simulink model "SDV"  (R2017a)
settings: Solver=ode4  StartTime=0.0  StopTime=100  FixedStep=0.01  RelTol=1e-3
values from neighbouring files (symbols this model uses):
  b = 0.1    [sdv_motion_control.m]
  d_stpms = 0.2    [sdv_motion_control.m]
  J = 0.01    [sdv_motion_control.m]
  ka = 5.0    (= 5)    [sdv_motion_control.m]
  kb = 5.0    (= 5)    [sdv_motion_control.m]
  ke = 0.1    [sdv_motion_control.m]
  kt = 0.1    [sdv_motion_control.m]
  L = 0.5    [sdv_motion_control.m]
  mod_engranajes = 0.5    [sdv_motion_control.m]
  R = 1.0    (= 1)    [sdv_motion_control.m]
  r_rueda = 0.025    [sdv_motion_control.m]
  thresh_ang = 30*pi/180    (= 0.523598775598)    [sdv_motion_control.m]
  v_max = 18    [sdv_motion_control.m]
libraries: simulink x3
settings Model: Creator=Usuario  LastModifiedBy=Usuario

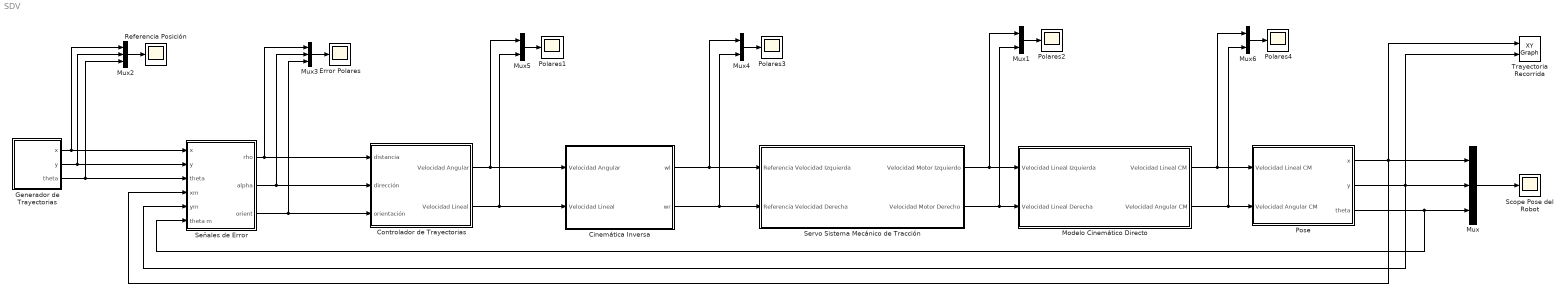
== system SDV ==
  Cinemática Inversa : Subsystem
  Controlador de Trayectorias : Subsystem
  Error Polares : Scope
  Generador de Trayectorias : Subsystem
  Modelo Cinemático Directo : Subsystem
  Mux : Mux  Inputs=3
  Mux{1,4..6} (4 alike) : Mux  Inputs=2
  Mux2 : Mux  Inputs=3
  Mux3 : Mux  Inputs=3
  Polares{1..4} (4 alike) : Scope
  Pose : Subsystem
  Referencia Posición : Scope
  Scope Pose del Robot : Scope
  Servo Sistema Mecánico de Tracción : Subsystem
  Señales de Error : Subsystem
  Trayectoria Recorrida : simulink/Sinks/XY Graph  xmin=-25  xmax=25  ymin=-25  ymax=25  st=-1
  wires:
  Mux/1 -> Scope Pose del Robot/1
  Pose/2(y) -> Trayectoria Recorrida/2, Mux/2, Señales de Error/5(ym)
  Pose/3(theta) -> Mux/3, Señales de Error/6(theta m)
  Pose/1(x) -> Trayectoria Recorrida/1, Mux/1, Señales de Error/4(xm)
  Mux2/1 -> Referencia Posición/1
  Mux3/1 -> Error Polares/1
  Mux5/1 -> Polares1/1
  Controlador de Trayectorias/1(Velocidad Angular) -> Mux5/1, Cinemática Inversa/1(Velocidad Angular)
  Señales de Error/2(alpha) -> Mux3/2, Controlador de Trayectorias/2(dirección)
  Señales de Error/1(rho) -> Mux3/1, Controlador de Trayectorias/1(distancia)
  Generador de Trayectorias/1(x) -> Mux2/1, Señales de Error/1(x)
  Generador de Trayectorias/2(y) -> Mux2/2, Señales de Error/2(y)
  Generador de Trayectorias/3(theta) -> Mux2/3, Señales de Error/3(theta)
  Señales de Error/3(orient) -> Controlador de Trayectorias/3(orientación), Mux3/3
  Controlador de Trayectorias/2(Velocidad Lineal) -> Mux5/2, Cinemática Inversa/2(Velocidad Lineal)
  Servo Sistema Mecánico de Tracción/1(Velocidad Motor Izquierdo) -> Mux1/1, Modelo Cinemático Directo/1(Velocidad Lineal Izquierda)
  Servo Sistema Mecánico de Tracción/2(Velocidad Motor Derecho) -> Mux1/2, Modelo Cinemático Directo/2(Velocidad Lineal Derecha)
  Mux1/1 -> Polares2/1
  Cinemática Inversa/1(wl) -> Mux4/1, Servo Sistema Mecánico de Tracción/1(Referencia Velocidad Izquierda)
  Mux4/1 -> Polares3/1
  Cinemática Inversa/2(wr) -> Mux4/2, Servo Sistema Mecánico de Tracción/2(Referencia Velocidad Derecha)
  Modelo Cinemático Directo/2(Velocidad Angular CM) -> Mux6/2, Pose/2(Velocidad Angular CM)
  Modelo Cinemático Directo/1(Velocidad Lineal CM) -> Mux6/1, Pose/1(Velocidad Lineal CM)
  Mux6/1 -> Polares4/1

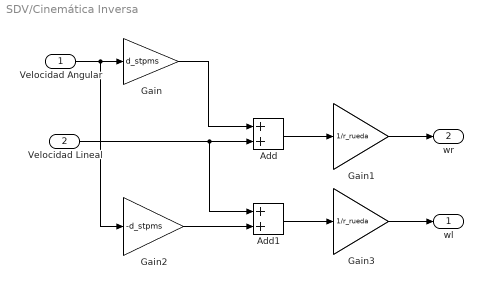
== system SDV/Cinemática Inversa ==
  Velocidad Angular : Inport
  Velocidad Lineal : Inport  Port=2
  Add : Sum
  Add1 : Sum
  Gain : Gain  Gain=d_stpms
  Gain1 : Gain  Gain=1/r_rueda
  Gain2 : Gain  Gain=-d_stpms
  Gain3 : Gain  Gain=1/r_rueda
  wl : Outport
  wr : Outport  Port=2
  wires:
  Velocidad Angular/1 -> Gain2/1, Gain/1
  Gain/1 -> Add/1
  Add/1 -> Gain1/1
  Gain1/1 -> wr/1
  Gain2/1 -> Add1/2
  Velocidad Lineal/1 -> Add1/1, Add/2
  Add1/1 -> Gain3/1
  Gain3/1 -> wl/1

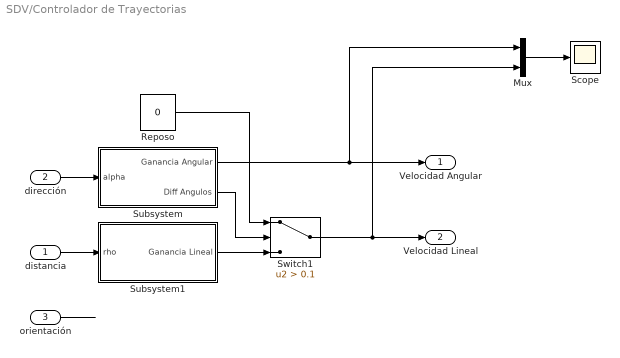
== system SDV/Controlador de Trayectorias ==
  distancia : Inport
  dirección : Inport  Port=2
  orientación : Inport  Port=3
  Mux : Mux  Inputs=2
  Reposo : Constant  Value=0
  Scope : Scope
  Subsystem : Subsystem
  Subsystem1 : Subsystem
  Switch1 : Switch  Criteria=u2 > Threshold  Threshold=0.1
  Velocidad Angular : Outport
  Velocidad Lineal : Outport  Port=2
  wires:
  dirección/1 -> Subsystem/1(alpha)
  distancia/1 -> Subsystem1/1(rho)
  Subsystem1/1(Ganancia Lineal) -> Switch1/3
  Reposo/1 -> Switch1/1
  Subsystem/2(Diff Angulos) -> Switch1/2
  Switch1/1 -> Mux/2, Velocidad Lineal/1
  Subsystem/1(Ganancia Angular) -> Mux/1, Velocidad Angular/1
  orientación/1 -> ?
  Mux/1 -> Scope/1

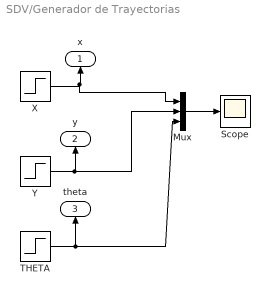
== system SDV/Generador de Trayectorias ==
  Mux : Mux  Inputs=3
  Scope : Scope
  THETA : Step  Time=0  After=0  SampleTime=0
  X : Step  Time=0  SampleTime=0
  Y : Step  Time=0  SampleTime=0
  x : Outport
  y : Outport  Port=2
  theta : Outport  Port=3
  wires:
  Y/1 -> y/1, Mux/2
  X/1 -> Mux/1, x/1
  THETA/1 -> Mux/3, theta/1
  Mux/1 -> Scope/1

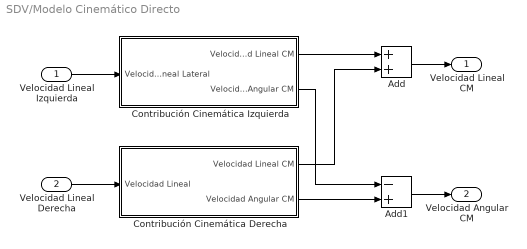
== system SDV/Modelo Cinemático Directo ==
  Velocidad Lineal Izquierda : Inport
  Velocidad Lineal Derecha : Inport  Port=2
  Add : Sum
  Add1 : Sum  Inputs=-+
  Contribución Cinemática Derecha : Subsystem
  Contribución Cinemática Izquierda : Subsystem
  Velocidad Lineal CM : Outport
  Velocidad Angular CM : Outport  Port=2
  wires:
  Velocidad Lineal Derecha/1 -> Contribución Cinemática Derecha/1(Velocidad Lineal)
  Velocidad Lineal Izquierda/1 -> Contribución Cinemática Izquierda/1(Velocidad Lineal Lateral)
  Add/1 -> Velocidad Lineal CM/1
  Add1/1 -> Velocidad Angular CM/1
  Contribución Cinemática Izquierda/2(Velocidad Angular CM) -> Add1/1
  Contribución Cinemática Derecha/2(Velocidad Angular CM) -> Add1/2
  Contribución Cinemática Derecha/1(Velocidad Lineal CM) -> Add/2
  Contribución Cinemática Izquierda/1(Velocidad Lineal CM) -> Add/1

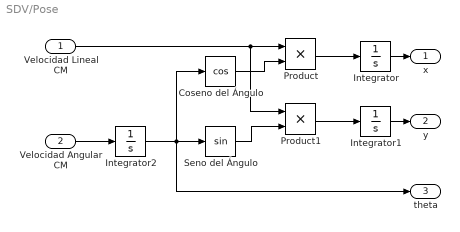
== system SDV/Pose ==
  Velocidad Lineal CM : Inport
  Velocidad Angular CM : Inport  Port=2
  Coseno del Ángulo : Trigonometry  Operator=cos
  Integrator : Integrator
  Integrator1 : Integrator
  Integrator2 : Integrator
  Product : Product
  Product1 : Product
  Seno del Ángulo : Trigonometry
  x : Outport
  y : Outport  Port=2
  theta : Outport  Port=3
  wires:
  Coseno del Ángulo/1 -> Product/2
  Integrator/1 -> x/1
  Product/1 -> Integrator/1
  Product1/1 -> Integrator1/1
  Integrator1/1 -> y/1
  Seno del Ángulo/1 -> Product1/2
  Velocidad Lineal CM/1 -> Product1/1, Product/1
  Velocidad Angular CM/1 -> Integrator2/1
  Integrator2/1 -> theta/1, Seno del Ángulo/1, Coseno del Ángulo/1

== system SDV/Servo Sistema Mecánico de Tracción ==
  Referencia Velocidad Izquierda : Inport
  Referencia Velocidad Derecha : Inport  Port=2
  Servo Controlador ESCON 50/5 Derecho : Subsystem
  Servo Controlador ESCON 50/5 Izquierdo : Subsystem
  Velocidad Motor Izquierdo : Outport
  Velocidad Motor Derecho : Outport  Port=2
  wires:
  Referencia Velocidad Izquierda/1 -> Servo Controlador ESCON 50/5 Izquierdo/1(Referencia Velocidad Izquierda)
  Referencia Velocidad Derecha/1 -> Servo Controlador ESCON 50/5 Derecho/1(Referencia Velocidad Derecha)
  Servo Controlador ESCON 50/5 Izquierdo/1(Velocidad Izquierda) -> Velocidad Motor Izquierdo/1
  Servo Controlador ESCON 50/5 Derecho/1(Velocidad Izquierda) -> Velocidad Motor Derecho/1

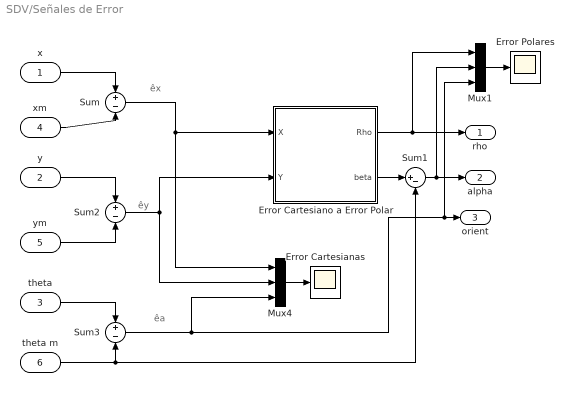
== system SDV/Señales de Error ==
  note: êa
  note: êy
  note: êx
  x : Inport
  y : Inport  Port=2
  theta : Inport  Port=3
  xm : Inport  Port=4
  ym : Inport  Port=5
  theta m : Inport  Port=6
  Error Cartesianas : Scope
  Error Polares : Scope
  Error Cartesiano a Error Polar : Subsystem
  Mux1 : Mux  Inputs=3
  Mux4 : Mux  Inputs=3
  Sum : Sum  Inputs=+-
  Sum1 : Sum  Inputs=|+-
  Sum2 : Sum  Inputs=+-
  Sum3 : Sum  Inputs=+-
  rho : Outport
  alpha : Outport  Port=2
  orient : Outport  Port=3
  wires:
  Sum/1 -> Mux4/1, Error Cartesiano a Error Polar/1(X)
  Sum2/1 -> Mux4/2, Error Cartesiano a Error Polar/2(Y)
  Error Cartesiano a Error Polar/1(Rho) -> Mux1/1, rho/1
  Mux4/1 -> Error Cartesianas/1
  Sum1/1 -> Mux1/2, alpha/1
  x/1 -> Sum/1
  y/1 -> Sum2/1
  xm/1 -> Sum/2
  ym/1 -> Sum2/2
  theta m/1 -> Sum1/2, Sum3/2
  theta/1 -> Sum3/1
  Sum3/1 -> Mux1/3, orient/1, Mux4/3
  Mux1/1 -> Error Polares/1
  Error Cartesiano a Error Polar/2(beta) -> Sum1/1

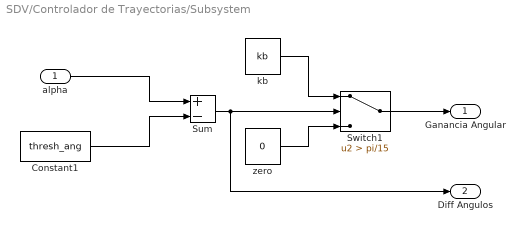
== system SDV/Controlador de Trayectorias/Subsystem ==
  alpha : Inport
  Constant1 : Constant  Value=thresh_ang
  Sum : Sum  Inputs=+-
  Switch1 : Switch  Criteria=u2 > Threshold  Threshold=pi/15
  "kb " : Constant  Value=kb
  zero : Constant  Value=0
  Ganancia Angular : Outport
  Diff Angulos : Outport  Port=2
  wires:
  Switch1/1 -> Ganancia Angular/1
  alpha/1 -> Sum/1
  Constant1/1 -> Sum/2
  "kb "/1 -> Switch1/1
  zero/1 -> Switch1/3
  Sum/1 -> Diff Angulos/1, Switch1/2

== system SDV/Controlador de Trayectorias/Subsystem1 ==
  rho : Inport
  Reposo : Constant  Value=0
  Switch : Switch  Criteria=u2 > Threshold  Threshold=0.1
  "ka " : Constant  Value=ka
  Ganancia Lineal : Outport
  wires:
  "ka "/1 -> Switch/1
  Switch/1 -> Ganancia Lineal/1
  rho/1 -> Switch/2
  Reposo/1 -> Switch/3

== system SDV/Modelo Cinemático Directo/Contribución Cinemática Derecha ==
  Velocidad Lineal : Inport
  Velcidad Lineal CM : Gain  Gain=0.5
  Velcidad Lineal CM1 : Gain  Gain=d_stpms/2
  Velocidad Lineal CM : Outport
  Velocidad Angular CM : Outport  Port=2
  wires:
  Velocidad Lineal/1 -> Velcidad Lineal CM1/1, Velcidad Lineal CM/1
  Velcidad Lineal CM/1 -> Velocidad Lineal CM/1
  Velcidad Lineal CM1/1 -> Velocidad Angular CM/1

== system SDV/Modelo Cinemático Directo/Contribución Cinemática Izquierda ==
  Velocidad Lineal Lateral : Inport
  Interpolación Lineal Angular : Gain  Gain=d_stpms/2
  Interpolación Lineal Lineal : Gain  Gain=0.5
  Velocidad Lineal CM : Outport
  Velocidad Angular CM : Outport  Port=2
  wires:
  Velocidad Lineal Lateral/1 -> Interpolación Lineal Angular/1, Interpolación Lineal Lineal/1
  Interpolación Lineal Lineal/1 -> Velocidad Lineal CM/1
  Interpolación Lineal Angular/1 -> Velocidad Angular CM/1

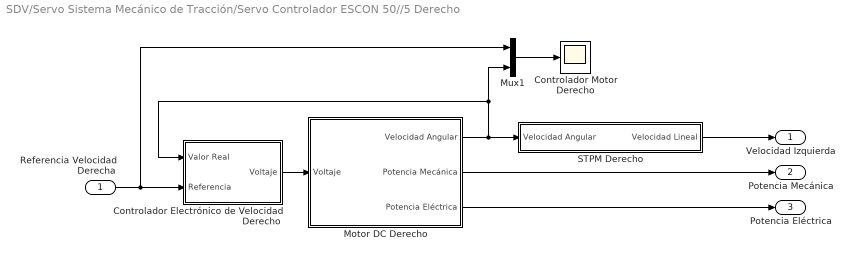
== system SDV/Servo Sistema Mecánico de Tracción/Servo Controlador ESCON 50//5 Derecho ==
  Referencia Velocidad Derecha : Inport
  Controlador Electrónico de Velocidad Derecho : Subsystem
  Controlador Motor Derecho : Scope
  Motor DC Derecho : Subsystem
  Mux1 : Mux  Inputs=2
  STPM Derecho : Subsystem
  Velocidad Izquierda : Outport
  Potencia Mecánica : Outport  Port=2
  Potencia Eléctrica : Outport  Port=3
  wires:
  Motor DC Derecho/1(Velocidad Angular) -> Mux1/2, Controlador Electrónico de Velocidad Derecho/1(Valor Real), STPM Derecho/1(Velocidad Angular)
  STPM Derecho/1(Velocidad Lineal) -> Velocidad Izquierda/1
  Controlador Electrónico de Velocidad Derecho/1(Voltaje) -> Motor DC Derecho/1("Voltaje ")
  Mux1/1 -> Controlador Motor Derecho/1
  Motor DC Derecho/2(Potencia Mecánica) -> Potencia Mecánica/1
  Motor DC Derecho/3(Potencia Eléctrica) -> Potencia Eléctrica/1
  Referencia Velocidad Derecha/1 -> Mux1/1, Controlador Electrónico de Velocidad Derecho/2(Referencia)

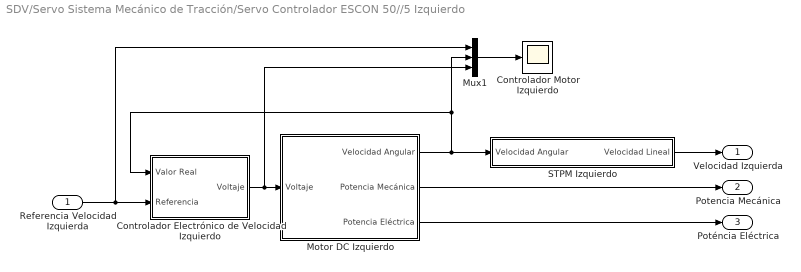
== system SDV/Servo Sistema Mecánico de Tracción/Servo Controlador ESCON 50//5 Izquierdo ==
  Referencia Velocidad Izquierda : Inport
  Controlador Electrónico de Velocidad Izquierdo : Subsystem
  Controlador Motor Izquierdo : Scope
  "Motor DC Izquierdo " : Subsystem
  Mux1 : Mux  Inputs=3
  STPM Izquierdo : Subsystem
  Velocidad Izquierda : Outport
  Potencia Mecánica : Outport  Port=2
  Poténcia Eléctrica : Outport  Port=3
  wires:
  Referencia Velocidad Izquierda/1 -> Mux1/1, Controlador Electrónico de Velocidad Izquierdo/2(Referencia)
  Controlador Electrónico de Velocidad Izquierdo/1(Voltaje) -> Mux1/3, "Motor DC Izquierdo "/1("Voltaje ")
  STPM Izquierdo/1(Velocidad Lineal) -> Velocidad Izquierda/1
  "Motor DC Izquierdo "/2(Potencia Mecánica) -> Potencia Mecánica/1
  "Motor DC Izquierdo "/3(Potencia Eléctrica) -> Poténcia Eléctrica/1
  Mux1/1 -> Controlador Motor Izquierdo/1
  "Motor DC Izquierdo "/1(Velocidad Angular) -> STPM Izquierdo/1(Velocidad Angular), Mux1/2, Controlador Electrónico de Velocidad Izquierdo/1(Valor Real)

== system SDV/Señales de Error/Error Cartesiano a Error Polar ==
  X : Inport
  Y : Inport  Port=2
  Error Cartesianas : Scope
  Mux4 : Mux  Inputs=3
  Norma Euclidea : Subsystem
  Ángulo : Trigonometry  Operator=atan2
  Rho : Outport
  beta : Outport  Port=2
  wires:
  X/1 -> Mux4/2, Ángulo/2, Norma Euclidea/1(x)
  Y/1 -> Mux4/1, Ángulo/1, Norma Euclidea/2(y)
  Ángulo/1 -> Mux4/3, beta/1
  Norma Euclidea/1(rho) -> Rho/1
  Mux4/1 -> Error Cartesianas/1

== system SDV/Servo Sistema Mecánico de Tracción/Servo Controlador ESCON 50//5 Derecho/Controlador Electrónico de Velocidad Derecho ==
  Valor Real : Inport
  Referencia : Inport  Port=2
  PID Controller : simulink/Continuous/PID Controller  Controller=PID  TimeDomain=Continuous-time  SampleTime=-1  IntegratorMethod=Forward Euler  FilterMethod=Forward Euler  Form=Parallel  UseFilter=on  ControllerParametersSource=internal  P=2.10211370234041  I=6.4024299686163  D=0.114524010077378  N=42.1465473300371  InitialConditionSource=internal  InitialConditionForIntegrator=0  InitialConditionForFilter=0  ExternalReset=none  LimitOutput=off  UpperSaturationLimit=inf  LowerSaturationLimit=-inf  LinearizeAsGain=on  AntiWindupMode=none  Kb=1  TrackingMode=off  Kt=1  PParamMin=[]  PParamMax=[]  IParamMin=[]  IParamMax=[]  DParamMin=[]  DParamMax=[]  NParamMin=[]  NParamMax=[]  KbParamMin=[]  KbParamMax=[]  KtParamMin=[]  KtParamMax=[]  POutMin=[]  POutMax=[]  IOutMin=[]  IOutMax=[]  DOutMin=[]  DOutMax=[]  NOutMin=[]  NOutMax=[]  KbOutMin=[]  KbOutMax=[]  KtOutMin=[]  KtOutMax=[]  IntegratorOutMin=[]  IntegratorOutMax=[]  FilterOutMin=[]  FilterOutMax=[]  SumOutMin=[]  SumOutMax=[]  SumI1OutMin=[]  SumI1OutMax=[]  SumI2OutMin=[]  SumI2OutMax=[]  SumI3OutMin=[]  SumI3OutMax=[]  SumDOutMin=[]  SumDOutMax=[]  SaturationOutMin=[]  SaturationOutMax=[]  IntegratorContinuousStateAttributes=''  IntegratorStateMustResolveToSignalObject=off  IntegratorRTWStateStorageClass=Auto  FilterContinuousStateAttributes=''  FilterStateMustResolveToSignalObject=off  FilterRTWStateStorageClass=Auto  DifferentiatorICPrevScaledInput=0  DifferentiatorOutMin=[]  DifferentiatorOutMax=[]  InitialConditionSetting=State (most efficient)
  Saturation : Saturate  UpperLimit=v_max  LowerLimit=-v_max
  Sum : Sum  Inputs=|+-
  Valor Digital : Gain
  Voltaje Motor : Gain
  Voltaje : Outport
  wires:
  Voltaje Motor/1 -> Saturation/1
  Valor Real/1 -> Sum/2
  PID Controller/1 -> Valor Digital/1
  Sum/1 -> PID Controller/1
  Referencia/1 -> Sum/1
  Valor Digital/1 -> Voltaje Motor/1
  Saturation/1 -> Voltaje/1

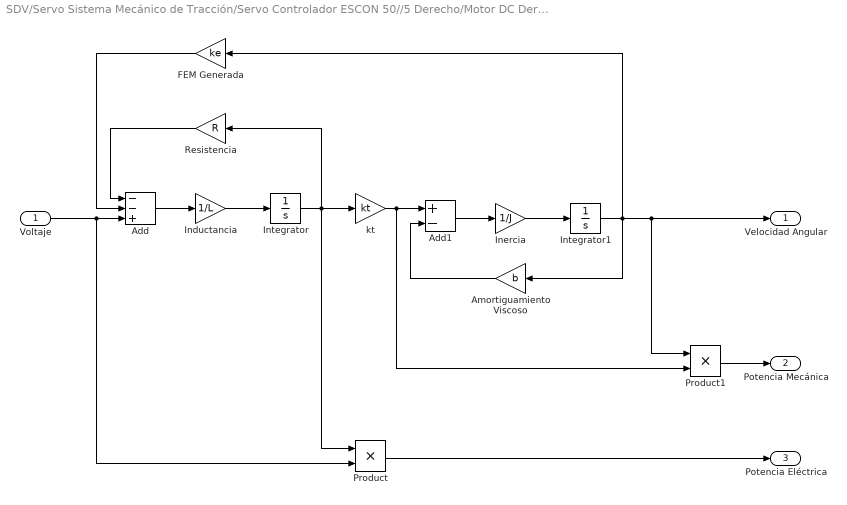
== system SDV/Servo Sistema Mecánico de Tracción/Servo Controlador ESCON 50//5 Derecho/Motor DC Derecho ==
  "Voltaje " : Inport
  Add : Sum  Inputs=--+
  Add1 : Sum  Inputs=+-
  Amortiguamiento Viscoso : Gain  Gain=b
  FEM Generada : Gain  Gain=ke
  Inductancia : Gain  Gain=1/L
  Inercia : Gain  Gain=1/J
  Integrator : Integrator
  Integrator1 : Integrator
  Product : Product
  Product1 : Product
  "Resistencia " : Gain  Gain=R
  kt : Gain  Gain=kt
  Velocidad Angular : Outport
  Potencia Mecánica : Outport  Port=2
  Potencia Eléctrica : Outport  Port=3
  wires:
  Amortiguamiento Viscoso/1 -> Add1/2
  FEM Generada/1 -> Add/2
  "Voltaje "/1 -> Product/2, Add/3
  Inductancia/1 -> Integrator/1
  Integrator/1 -> Product/1, "Resistencia "/1, kt/1
  kt/1 -> Product1/2, Add1/1
  Inercia/1 -> Integrator1/1
  Add1/1 -> Inercia/1
  Integrator1/1 -> Product1/1, Velocidad Angular/1, FEM Generada/1, Amortiguamiento Viscoso/1
  Add/1 -> Inductancia/1
  "Resistencia "/1 -> Add/1
  Product/1 -> Potencia Eléctrica/1
  Product1/1 -> Potencia Mecánica/1

== system SDV/Servo Sistema Mecánico de Tracción/Servo Controlador ESCON 50//5 Derecho/STPM Derecho ==
  Velocidad Angular : Inport
  Módulo de Engranajes : Gain  Gain=mod_engranajes
  Radio Rueda : Gain  Gain=r_rueda
  Velocidad Lineal : Outport
  wires:
  Módulo de Engranajes/1 -> Radio Rueda/1
  Velocidad Angular/1 -> Módulo de Engranajes/1
  Radio Rueda/1 -> Velocidad Lineal/1

== system SDV/Servo Sistema Mecánico de Tracción/Servo Controlador ESCON 50//5 Izquierdo/Controlador Electrónico de Velocidad Izquierdo ==
  Valor Real : Inport
  Referencia : Inport  Port=2
  PID Controller : simulink/Continuous/PID Controller  Controller=PID  TimeDomain=Continuous-time  SampleTime=-1  IntegratorMethod=Forward Euler  FilterMethod=Forward Euler  Form=Parallel  UseFilter=on  ControllerParametersSource=internal  P=2.10211370234041  I=6.4024299686163  D=0.114524010077378  N=42.1465473300371  InitialConditionSource=internal  InitialConditionForIntegrator=0  InitialConditionForFilter=0  ExternalReset=none  LimitOutput=off  UpperSaturationLimit=inf  LowerSaturationLimit=-inf  LinearizeAsGain=on  AntiWindupMode=none  Kb=1  TrackingMode=off  Kt=1  PParamMin=[]  PParamMax=[]  IParamMin=[]  IParamMax=[]  DParamMin=[]  DParamMax=[]  NParamMin=[]  NParamMax=[]  KbParamMin=[]  KbParamMax=[]  KtParamMin=[]  KtParamMax=[]  POutMin=[]  POutMax=[]  IOutMin=[]  IOutMax=[]  DOutMin=[]  DOutMax=[]  NOutMin=[]  NOutMax=[]  KbOutMin=[]  KbOutMax=[]  KtOutMin=[]  KtOutMax=[]  IntegratorOutMin=[]  IntegratorOutMax=[]  FilterOutMin=[]  FilterOutMax=[]  SumOutMin=[]  SumOutMax=[]  SumI1OutMin=[]  SumI1OutMax=[]  SumI2OutMin=[]  SumI2OutMax=[]  SumI3OutMin=[]  SumI3OutMax=[]  SumDOutMin=[]  SumDOutMax=[]  SaturationOutMin=[]  SaturationOutMax=[]  IntegratorContinuousStateAttributes=''  IntegratorStateMustResolveToSignalObject=off  IntegratorRTWStateStorageClass=Auto  FilterContinuousStateAttributes=''  FilterStateMustResolveToSignalObject=off  FilterRTWStateStorageClass=Auto  DifferentiatorICPrevScaledInput=0  DifferentiatorOutMin=[]  DifferentiatorOutMax=[]  InitialConditionSetting=State (most efficient)
  Saturation : Saturate  UpperLimit=v_max  LowerLimit=-v_max
  Sum : Sum  Inputs=-|+
  Valor Digital : Gain
  Voltaje Motor : Gain
  Voltaje : Outport
  wires:
  Voltaje Motor/1 -> Saturation/1
  Valor Real/1 -> Sum/1
  PID Controller/1 -> Valor Digital/1
  Sum/1 -> PID Controller/1
  Valor Digital/1 -> Voltaje Motor/1
  Saturation/1 -> Voltaje/1
  Referencia/1 -> Sum/2

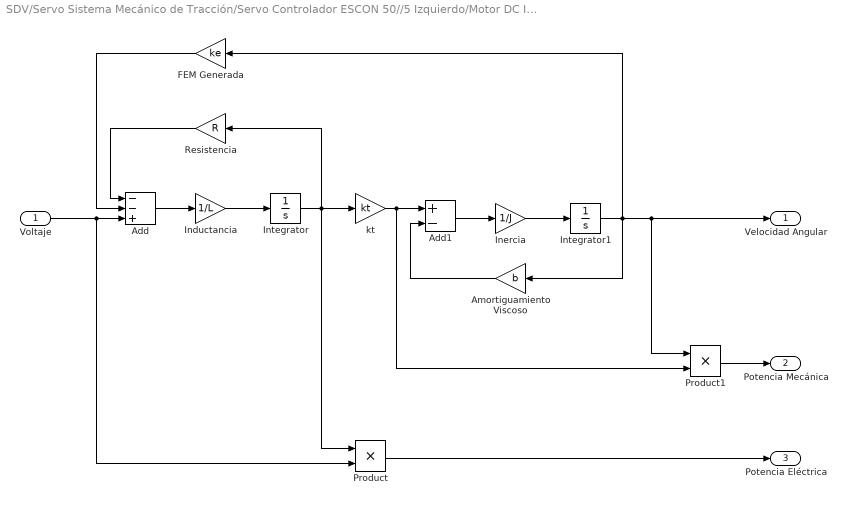
== system SDV/Servo Sistema Mecánico de Tracción/Servo Controlador ESCON 50//5 Izquierdo/Motor DC Izquierdo  ==
  "Voltaje " : Inport
  Add : Sum  Inputs=--+
  Add1 : Sum  Inputs=+-
  Amortiguamiento Viscoso : Gain  Gain=b
  FEM Generada : Gain  Gain=ke
  Inductancia : Gain  Gain=1/L
  Inercia : Gain  Gain=1/J
  Integrator : Integrator
  Integrator1 : Integrator
  Product : Product
  Product1 : Product
  "Resistencia " : Gain  Gain=R
  kt : Gain  Gain=kt
  Velocidad Angular : Outport
  Potencia Mecánica : Outport  Port=2
  Potencia Eléctrica : Outport  Port=3
  wires:
  Amortiguamiento Viscoso/1 -> Add1/2
  FEM Generada/1 -> Add/2
  "Voltaje "/1 -> Product/2, Add/3
  Inductancia/1 -> Integrator/1
  Integrator/1 -> Product/1, "Resistencia "/1, kt/1
  kt/1 -> Product1/2, Add1/1
  Inercia/1 -> Integrator1/1
  Add1/1 -> Inercia/1
  Integrator1/1 -> Product1/1, Velocidad Angular/1, FEM Generada/1, Amortiguamiento Viscoso/1
  Add/1 -> Inductancia/1
  "Resistencia "/1 -> Add/1
  Product/1 -> Potencia Eléctrica/1
  Product1/1 -> Potencia Mecánica/1

== system SDV/Servo Sistema Mecánico de Tracción/Servo Controlador ESCON 50//5 Izquierdo/STPM Izquierdo ==
  Velocidad Angular : Inport
  Módulo de Engranajes : Gain  Gain=mod_engranajes
  Radio Rueda : Gain  Gain=r_rueda
  Velocidad Lineal : Outport
  wires:
  Módulo de Engranajes/1 -> Radio Rueda/1
  Velocidad Angular/1 -> Módulo de Engranajes/1
  Radio Rueda/1 -> Velocidad Lineal/1

== system SDV/Señales de Error/Error Cartesiano a Error Polar/Norma Euclidea ==
  x : Inport
  y : Inport  Port=2
  Add : Sum
  Sqrt : Sqrt  SaturateOnIntegerOverflow=on
  x2 : Product
  y2 : Product
  rho : Outport
  wires:
  x/1 -> x2/2, x2/1
  y/1 -> y2/2, y2/1
  Sqrt/1 -> rho/1
  y2/1 -> Add/2
  Add/1 -> Sqrt/1
  x2/1 -> Add/1
